simulink library "cps_lib_v2"  (R2012b)
settings: Solver=ode45  StartTime=0.0  StopTime=10.0  RelTol=1e-3
undefined symbols (not defined in the file or in its folder): block_height, block_mass, block_width, board_vpos, ini_block_hpos, ini_block_vpos, nozzle_radius
libraries: fl_lib x88, nesl_utility x7, vrlib x5, cps_physics_lib x3
settings Model: Creator=pmosterm  LastModifiedBy=pmosterm

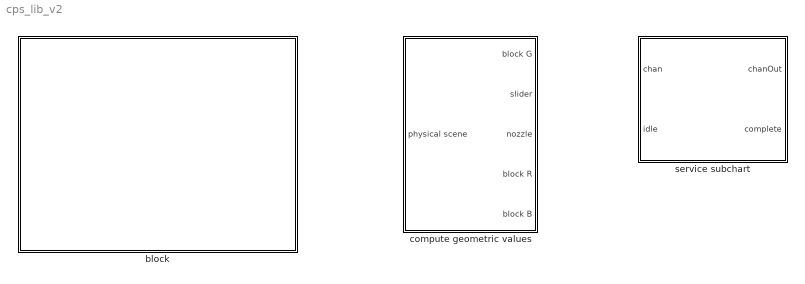
== system cps_lib_v2 ==
  block : Subsystem  mask{ini_block_vpos=ini_block_vpos, ini_block_hpos=ini_block_hpos}
      mask prompts: ini_block_vpos "Initial vertical block position"; ini_block_hpos "Initial horizontal block position"
      mask Display: image(imread('images\geo_ton_blocks_274x212.jpg'));
  compute geometric values : Subsystem
  service subchart : Stateflow chart  TreatAsAtomicUnit=on

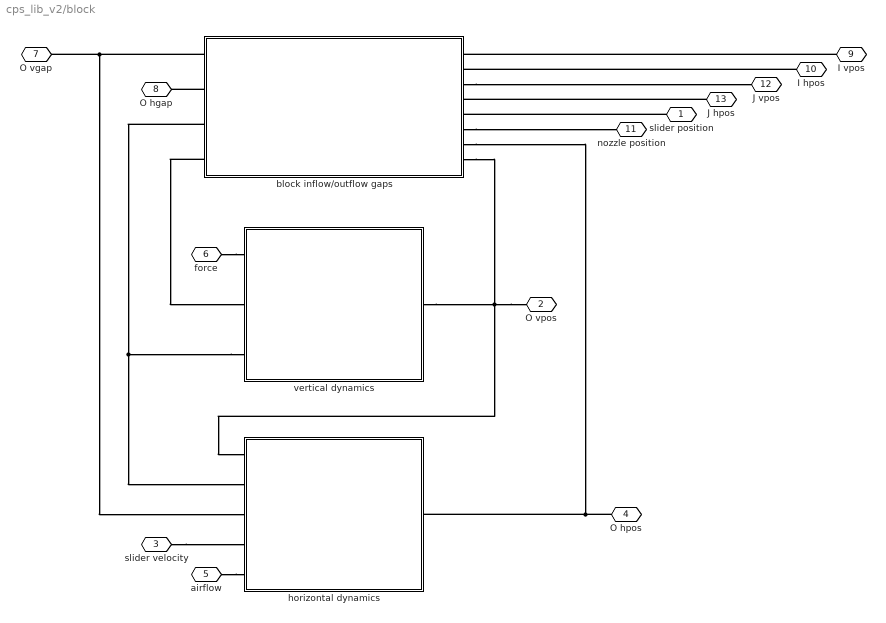
== system cps_lib_v2/block ==
  block inflow/outflow gaps : Subsystem
      settings: OpenFcn=open_system(gcb,'force');
      mask Display: image(imread('images\geo_ton_gaps_256x130.jpg'));
  horizontal dynamics : Subsystem
      settings: OpenFcn=open_system(gcb,'force');
      mask Display: image(imread('images\geo_ton_block_horizontal_176x149.jpg'));
  vertical dynamics : Subsystem
      settings: OpenFcn=open_system(gcb,'force');
      mask Display: image(imread('images\geo_ton_block_vertical_176x150.jpg'));
  slider position : PMIOPort  Port=1  Side=Left
  O vpos : PMIOPort  Port=2  Side=Right
  slider velocity : PMIOPort  Port=3  Side=Left
  O hpos : PMIOPort  Port=4  Side=Right
  airflow : PMIOPort  Port=5  Side=Left
  force : PMIOPort  Port=6  Side=Left
  O vgap : PMIOPort  Port=7  Side=Left
  O hgap : PMIOPort  Port=8  Side=Left
  I vpos : PMIOPort  Port=9  Side=Right
  I hpos : PMIOPort  Port=10  Side=Right
  nozzle position : PMIOPort  Port=11  Side=Left
  J vpos : PMIOPort  Port=12  Side=Right
  J hpos : PMIOPort  Port=13  Side=Right
  connections:
  block inflow/outflow gaps/LConn6 -- nozzle position/RConn1
  slider position/RConn1 -- block inflow/outflow gaps/LConn5
  I hpos/RConn1 -- block inflow/outflow gaps/LConn2
  I vpos/RConn1 -- block inflow/outflow gaps/LConn1
  block inflow/outflow gaps/RConn2 -- O hgap/RConn1
  block inflow/outflow gaps/RConn4 -- vertical dynamics/LConn2
  force/RConn1 -- vertical dynamics/LConn1
  vertical dynamics/LConn3 -- horizontal dynamics/LConn2 -- block inflow/outflow gaps/RConn3
  airflow/RConn1 -- horizontal dynamics/LConn5
  block inflow/outflow gaps/RConn1 -- horizontal dynamics/LConn3 -- O vgap/RConn1
  O vpos/RConn1 -- block inflow/outflow gaps/LConn8 -- horizontal dynamics/LConn1 -- vertical dynamics/RConn1
  horizontal dynamics/RConn1 -- block inflow/outflow gaps/LConn7 -- O hpos/RConn1
  slider velocity/RConn1 -- horizontal dynamics/LConn4
  block inflow/outflow gaps/LConn3 -- J vpos/RConn1
  J hpos/RConn1 -- block inflow/outflow gaps/LConn4

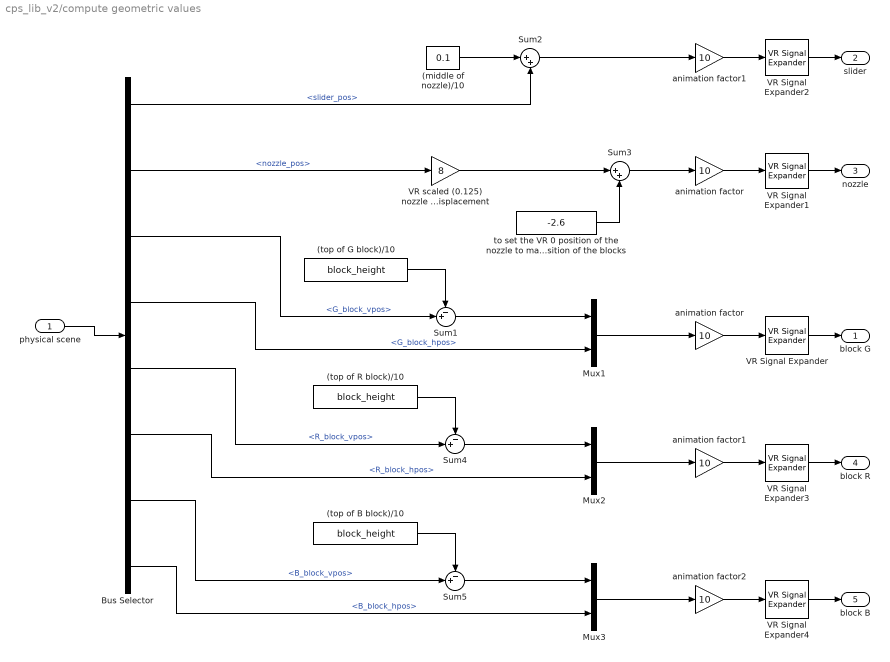
== system cps_lib_v2/compute geometric values ==
  physical scene : Inport  OutDataTypeStr=Bus: slBusGeometry
  " animation factor" : Gain  Gain=10
  " animation factor1" : Gain  Gain=10
  (middle of nozzle)/10 : Constant  Value=0.1
  (top of B block)/10 : Constant  Value=block_height
  (top of G block)/10 : Constant  Value=block_height
  (top of R block)/10 : Constant  Value=block_height
  Bus Selector : BusSelector  OutputSignals=slider_pos,nozzle_pos,G_block_vpos,G_block_hpos,R_block_vpos,R_block_hpos,B_block_vpos,B_block_hpos
  Mux1 : Mux  Inputs=2
  Mux2 : Mux  Inputs=2
  Mux3 : Mux  Inputs=2
  Sum1 : Sum  Inputs=-+|
  Sum2 : Sum  Inputs=|++
  Sum3 : Sum  Inputs=|++
  Sum4 : Sum  Inputs=-+|
  Sum5 : Sum  Inputs=-+|
  VR Signal Expander : vrlib/VR Signal Expander  outwidth=3  outidx=[2 3]
  VR Signal Expander1 : vrlib/VR Signal Expander  outwidth=3  outidx=[2]
  VR Signal Expander2 : vrlib/VR Signal Expander  outwidth=3  outidx=[3]
  VR Signal Expander3 : vrlib/VR Signal Expander  outwidth=3  outidx=[2 3]
  VR Signal Expander4 : vrlib/VR Signal Expander  outwidth=3  outidx=[2 3]
  VR scaled (0.125) nozzle displacement : Gain  Gain=8
  animation factor : Gain  Gain=10
  animation factor1 : Gain  Gain=10
  animation factor2 : Gain  Gain=10
  "to set the VR 0 position of the nozzle to match up with the VR 0 position of the blocks " : Constant  Value=-2.6
  block G : Outport
  slider : Outport  Port=2
  nozzle : Outport  Port=3
  block R : Outport  Port=4
  block B : Outport  Port=5
  wires:
  " animation factor"/1 -> VR Signal Expander1/1
  (middle of nozzle)/10/1 -> Sum2/1
  Bus Selector/1 -> Sum2/2  "<slider_pos>"
  animation factor/1 -> VR Signal Expander/1
  Mux1/1 -> animation factor/1
  Sum2/1 -> " animation factor1"/1
  VR Signal Expander2/1 -> slider/1
  VR Signal Expander1/1 -> nozzle/1
  Bus Selector/4 -> Mux1/2  "<G_block_hpos>"
  VR Signal Expander/1 -> block G/1
  " animation factor1"/1 -> VR Signal Expander2/1
  Sum3/1 -> " animation factor"/1
  Sum1/1 -> Mux1/1
  Bus Selector/3 -> Sum1/2  "<G_block_vpos>"
  Bus Selector/2 -> VR scaled (0.125) nozzle displacement/1  "<nozzle_pos>"
  physical scene/1 -> Bus Selector/1
  animation factor1/1 -> VR Signal Expander3/1
  Mux2/1 -> animation factor1/1
  VR Signal Expander3/1 -> block R/1
  Sum4/1 -> Mux2/1
  Bus Selector/6 -> Mux2/2  "<R_block_hpos>"
  Bus Selector/5 -> Sum4/2  "<R_block_vpos>"
  (top of G block)/10/1 -> Sum1/1
  (top of R block)/10/1 -> Sum4/1
  "to set the VR 0 position of the nozzle to match up with the VR 0 position of the blocks "/1 -> Sum3/2
  VR scaled (0.125) nozzle displacement/1 -> Sum3/1
  animation factor2/1 -> VR Signal Expander4/1
  Mux3/1 -> animation factor2/1
  VR Signal Expander4/1 -> block B/1
  Sum5/1 -> Mux3/1
  (top of B block)/10/1 -> Sum5/1
  Bus Selector/7 -> Sum5/2  "<B_block_vpos>"
  Bus Selector/8 -> Mux3/2  "<B_block_hpos>"

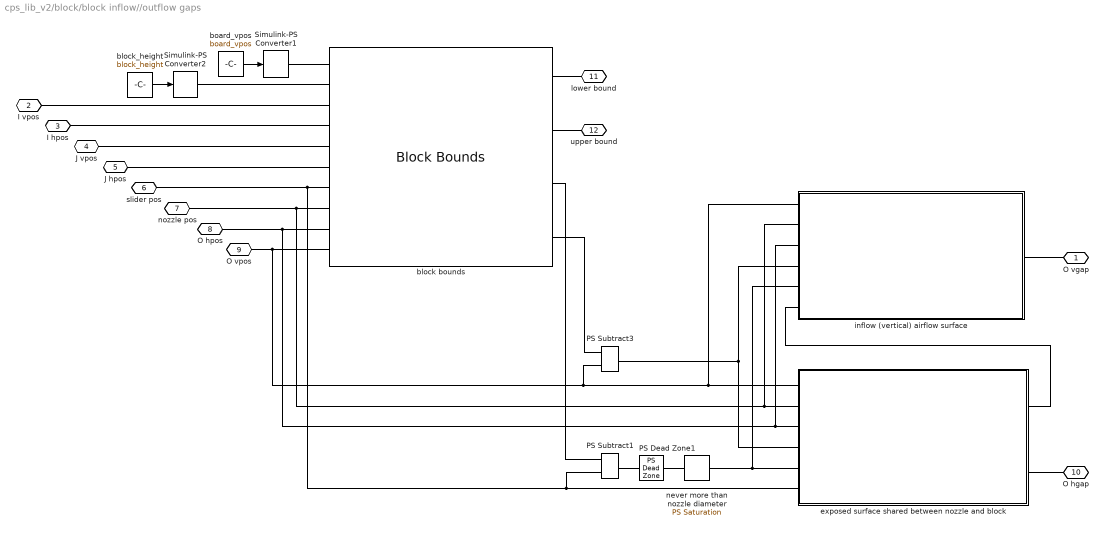
== system cps_lib_v2/block/block inflow//outflow gaps ==
  PS Dead Zone1 : fl_lib/Physical Signals/Nonlinear Operators/PS Dead Zone  upper_limit=0.5*block_width-nozzle_radius  lower_limit=-0.5*block_width+nozzle_radius  LocalVarLogging=[]
  PS Subtract1 : fl_lib/Physical Signals/Functions/PS Subtract  LocalVarLogging=[]
  PS Subtract3 : fl_lib/Physical Signals/Functions/PS Subtract  LocalVarLogging=[]
  Simulink-PS Converter1 : nesl_utility/Simulink-PS Converter  PhysicalDomain=network_engine_domain  LeftPortType=input  RightPortType=output  SubClassName=ps_input  PseudoPeriodic=off  Frequencies=[]  NoiseDistribution=none  NoiseParameters=[]  Unit=1  AffineConversion=off  InputFilterTimeConstant=.001  UdotUserProvided=[]  SimscapeFilterOrder=1  InputFiltering=off
  Simulink-PS Converter2 : nesl_utility/Simulink-PS Converter  PhysicalDomain=network_engine_domain  LeftPortType=input  RightPortType=output  SubClassName=ps_input  PseudoPeriodic=off  Frequencies=[]  NoiseDistribution=none  NoiseParameters=[]  Unit=1  AffineConversion=off  InputFilterTimeConstant=.001  UdotUserProvided=[]  SimscapeFilterOrder=1  InputFiltering=off
  block bounds : cps_physics_lib/Block Bounds  block_width=block_width m  nozzle_radius=nozzle_radius m  vmargin=1e-6 m  block_height_Log=off  board_vpos_Log=off  LocalVarNames=|block_height  LocalVarDescs=|Block Height  LocalVarLogging=[]
  block_height : Constant  Value=block_height
  board_vpos : Constant  Value=board_vpos
  exposed surface shared between nozzle and block : Subsystem
  inflow (vertical) airflow surface : Subsystem
  never more than nozzle diameter : fl_lib/Physical Signals/Nonlinear Operators/PS Saturation  upper_limit=2*nozzle_radius  lower_limit=-2*nozzle_radius  LocalVarLogging=[]
  O vgap : PMIOPort  Port=1  Side=Right
  I vpos : PMIOPort  Port=2  Side=Left
  I hpos : PMIOPort  Port=3  Side=Left
  J vpos : PMIOPort  Port=4  Side=Left
  J hpos : PMIOPort  Port=5  Side=Left
  slider pos : PMIOPort  Port=6  Side=Left
  nozzle pos : PMIOPort  Port=7  Side=Left
  O hpos : PMIOPort  Port=8  Side=Left
  O vpos : PMIOPort  Port=9  Side=Left
  O hgap : PMIOPort  Port=10  Side=Right
  lower bound : PMIOPort  Port=11  Side=Right
  upper bound : PMIOPort  Port=12  Side=Right
  wires:
  block_height/1 -> Simulink-PS Converter2/1
  board_vpos/1 -> Simulink-PS Converter1/1
  connections:
  PS Subtract1/RConn1 -- PS Dead Zone1/LConn1
  PS Dead Zone1/RConn1 -- never more than nozzle diameter/LConn1
  block bounds/LConn3 -- I vpos/RConn1
  never more than nozzle diameter/RConn1 -- exposed surface shared between nozzle and block/LConn5 -- inflow (vertical) airflow surface/LConn5
  block bounds/LConn4 -- I hpos/RConn1
  exposed surface shared between nozzle and block/LConn2 -- block bounds/LConn8 -- nozzle pos/RConn1 -- inflow (vertical) airflow surface/LConn2
  exposed surface shared between nozzle and block/LConn6 -- slider pos/RConn1 -- block bounds/LConn7 -- PS Subtract1/LConn2
  inflow (vertical) airflow surface/LConn1 -- exposed surface shared between nozzle and block/LConn1 -- block bounds/LConn10 -- O vpos/RConn1 -- PS Subtract3/LConn1
  inflow (vertical) airflow surface/LConn4 -- exposed surface shared between nozzle and block/LConn4 -- PS Subtract3/RConn1
  inflow (vertical) airflow surface/RConn1 -- O vgap/RConn1
  inflow (vertical) airflow surface/LConn3 -- exposed surface shared between nozzle and block/LConn3 -- block bounds/LConn9 -- O hpos/RConn1
  exposed surface shared between nozzle and block/RConn1 -- inflow (vertical) airflow surface/LConn6
  O hgap/RConn1 -- exposed surface shared between nozzle and block/RConn2
  block bounds/LConn5 -- J vpos/RConn1
  block bounds/LConn6 -- J hpos/RConn1
  block bounds/RConn1 -- lower bound/RConn1
  block bounds/RConn2 -- upper bound/RConn1
  block bounds/RConn4 -- PS Subtract3/LConn2
  block bounds/RConn3 -- PS Subtract1/LConn1
  Simulink-PS Converter2/RConn1 -- block bounds/LConn2
  Simulink-PS Converter1/RConn1 -- block bounds/LConn1

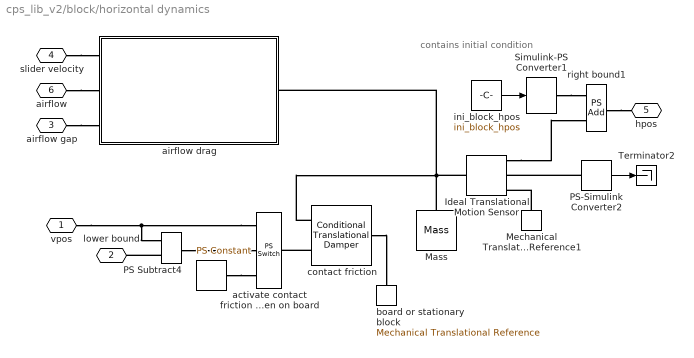
== system cps_lib_v2/block/horizontal dynamics ==
  note: contains initial condition
  " " : fl_lib/Physical Signals/Sources/PS Constant  constant=0  LocalVarLogging=[]
  Ideal Translational Motion Sensor : fl_lib/Mechanical/Mechanical Sensors/Ideal Translational Motion Sensor  offset=0 m  v_Log=off  f_Log=off  x_Log=off  LocalVarNames=|v|f|x  LocalVarDescs=|v|f|x  LocalVarLogging=[0 0 0]
  Mass : fl_lib/Mechanical/Translational Elements/Mass  mass=block_mass kg  initial_velocity=0 m/s  f_Log=off  LocalVarNames=|f  LocalVarDescs=|f  LocalVarLogging=0
  Mechanical Translational Reference1 : fl_lib/Mechanical/Translational Elements/Mechanical Translational Reference  f_Log=off  LocalVarNames=|f  LocalVarDescs=|f  LocalVarLogging=0
  PS Subtract4 : fl_lib/Physical Signals/Functions/PS Subtract  LocalVarLogging=[]
  PS-Simulink Converter2 : nesl_utility/PS-Simulink Converter  PhysicalDomain=network_engine_domain  LeftPortType=input  RightPortType=output  SubClassName=ps_output  PseudoPeriodic=off  Frequencies=[]  Unit=1  AffineConversion=off
  Simulink-PS Converter1 : nesl_utility/Simulink-PS Converter  PhysicalDomain=network_engine_domain  LeftPortType=input  RightPortType=output  SubClassName=ps_input  PseudoPeriodic=off  Frequencies=[]  NoiseDistribution=none  NoiseParameters=[]  Unit=1  AffineConversion=off  InputFilterTimeConstant=.001  UdotUserProvided=[]  SimscapeFilterOrder=1  InputFiltering=off
  Terminator2 : Terminator
  activate contact friction when on board : fl_lib/Physical Signals/Nonlinear Operators/PS Switch  Threshold=0  LocalVarLogging=[]
  airflow drag : Subsystem
  board or stationary block : fl_lib/Mechanical/Translational Elements/Mechanical Translational Reference  f_Log=off  LocalVarNames=|f  LocalVarDescs=|f  LocalVarLogging=0
  contact friction : cps_physics_lib/Conditional Translational Damper  D=100 N/(m/s)  th=1e-12  f_Log=off  v_Log=off  LocalVarNames=|f|v  LocalVarDescs=|f|v  LocalVarLogging=[0 0]
  ini_block_hpos : Constant  Value=ini_block_hpos
  right bound1 : fl_lib/Physical Signals/Functions/PS Add  LocalVarLogging=[]
  vpos : PMIOPort  Port=1  Side=Left
  lower bound : PMIOPort  Port=2  Side=Left
  airflow gap : PMIOPort  Port=3  Side=Left
  slider velocity : PMIOPort  Port=4  Side=Left
  hpos : PMIOPort  Port=5  Side=Right
  airflow : PMIOPort  Port=6  Side=Left
  wires:
  PS-Simulink Converter2/1 -> Terminator2/1
  ini_block_hpos/1 -> Simulink-PS Converter1/1
  connections:
  PS-Simulink Converter2/LConn1 -- Ideal Translational Motion Sensor/RConn2
  contact friction/LConn2 -- activate contact friction when on board/RConn1
  " "/RConn1 -- activate contact friction when on board/LConn3
  contact friction/RConn1 -- board or stationary block/LConn1
  PS Subtract4/RConn1 -- activate contact friction when on board/LConn2
  PS Subtract4/LConn2 -- lower bound/RConn1
  activate contact friction when on board/LConn1 -- vpos/RConn1 -- PS Subtract4/LConn1
  airflow gap/RConn1 -- airflow drag/LConn3
  airflow/RConn1 -- airflow drag/LConn2
  slider velocity/RConn1 -- airflow drag/LConn1
  Simulink-PS Converter1/RConn1 -- right bound1/LConn2
  Mechanical Translational Reference1/LConn1 -- Ideal Translational Motion Sensor/RConn1
  right bound1/RConn1 -- hpos/RConn1
  Ideal Translational Motion Sensor/RConn3 -- right bound1/LConn1
  Mass/LConn1 -- Ideal Translational Motion Sensor/LConn1 -- airflow drag/RConn1 -- contact friction/LConn1

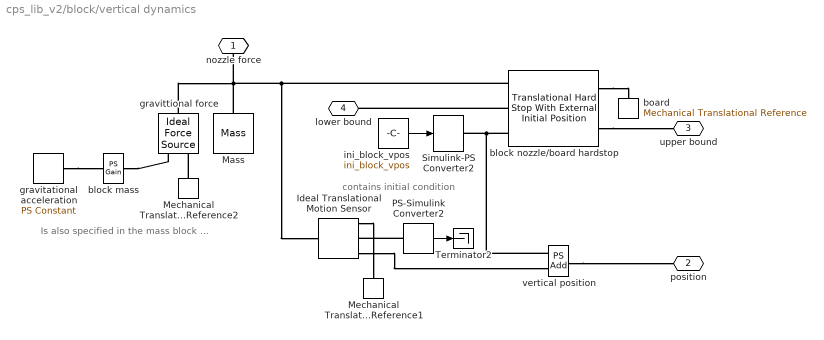
== system cps_lib_v2/block/vertical dynamics ==
  note: contains initial condition
  note: Is also specified in
      | the mass block ...
  Ideal Translational Motion Sensor : fl_lib/Mechanical/Mechanical Sensors/Ideal Translational Motion Sensor  offset=0 m  v_Log=off  f_Log=off  x_Log=off  LocalVarNames=|v|f|x  LocalVarDescs=|v|f|x  LocalVarLogging=[0 0 0]
  Mass : fl_lib/Mechanical/Translational Elements/Mass  mass=block_mass kg  initial_velocity=0 m/s  f_Log=off  LocalVarNames=|f  LocalVarDescs=|f  LocalVarLogging=0
  Mechanical Translational Reference1 : fl_lib/Mechanical/Translational Elements/Mechanical Translational Reference  f_Log=off  LocalVarNames=|f  LocalVarDescs=|f  LocalVarLogging=0
  Mechanical Translational Reference2 : fl_lib/Mechanical/Translational Elements/Mechanical Translational Reference  f_Log=off  LocalVarNames=|f  LocalVarDescs=|f  LocalVarLogging=0
  PS-Simulink Converter2 : nesl_utility/PS-Simulink Converter  PhysicalDomain=network_engine_domain  LeftPortType=input  RightPortType=output  SubClassName=ps_output  PseudoPeriodic=off  Frequencies=[]  Unit=1  AffineConversion=off
  Simulink-PS Converter2 : nesl_utility/Simulink-PS Converter  PhysicalDomain=network_engine_domain  LeftPortType=input  RightPortType=output  SubClassName=ps_input  PseudoPeriodic=off  Frequencies=[]  NoiseDistribution=none  NoiseParameters=[]  Unit=1  AffineConversion=off  InputFilterTimeConstant=.001  UdotUserProvided=[]  SimscapeFilterOrder=1  InputFiltering=off
  Terminator2 : Terminator
  block nozzle/board hardstop : cps_physics_lib/Translational Hard Stop With External Initial Position  stiff_up=3e4 N/m  stiff_low=1e5 N/m  D_up=450 N/(m/s)  D_low=450 N/(m/s)  f_Log=off  v_Log=off  x_Log=off  LocalVarNames=|f|v|x  LocalVarDescs=|f|v|x  LocalVarLogging=[0 0 0]
  block mass : fl_lib/Physical Signals/Functions/PS Gain  gain=block_mass  LocalVarLogging=[]
  board : fl_lib/Mechanical/Translational Elements/Mechanical Translational Reference  f_Log=off  LocalVarNames=|f  LocalVarDescs=|f  LocalVarLogging=0
  gravitational acceleration : fl_lib/Physical Signals/Sources/PS Constant  constant=-9.81  LocalVarLogging=[]
  gravittional force : fl_lib/Mechanical/Mechanical Sources/Ideal Force Source  v_Log=off  f_Log=off  LocalVarNames=|v|f  LocalVarDescs=|v|f  LocalVarLogging=[0 0]
  ini_block_vpos : Constant  Value=ini_block_vpos
  vertical position : fl_lib/Physical Signals/Functions/PS Add  LocalVarLogging=[]
  nozzle force : PMIOPort  Port=1  Side=Left
  position : PMIOPort  Port=2  Side=Right
  upper bound : PMIOPort  Port=3  Side=Left
  lower bound : PMIOPort  Port=4  Side=Left
  wires:
  PS-Simulink Converter2/1 -> Terminator2/1
  ini_block_vpos/1 -> Simulink-PS Converter2/1
  connections:
  PS-Simulink Converter2/LConn1 -- Ideal Translational Motion Sensor/RConn2
  Ideal Translational Motion Sensor/RConn3 -- vertical position/LConn2
  block nozzle/board hardstop/RConn2 -- upper bound/RConn1
  Simulink-PS Converter2/RConn1 -- block nozzle/board hardstop/LConn3 -- vertical position/LConn1
  block nozzle/board hardstop/RConn1 -- board/LConn1
  block nozzle/board hardstop/LConn2 -- lower bound/RConn1
  vertical position/RConn1 -- position/RConn1
  Ideal Translational Motion Sensor/RConn1 -- Mechanical Translational Reference1/LConn1
  nozzle force/RConn1 -- Mass/LConn1 -- gravittional force/LConn1 -- block nozzle/board hardstop/LConn1 -- Ideal Translational Motion Sensor/LConn1
  Mechanical Translational Reference2/LConn1 -- gravittional force/RConn2
  gravitational acceleration/RConn1 -- block mass/LConn1
  block mass/RConn1 -- gravittional force/RConn1

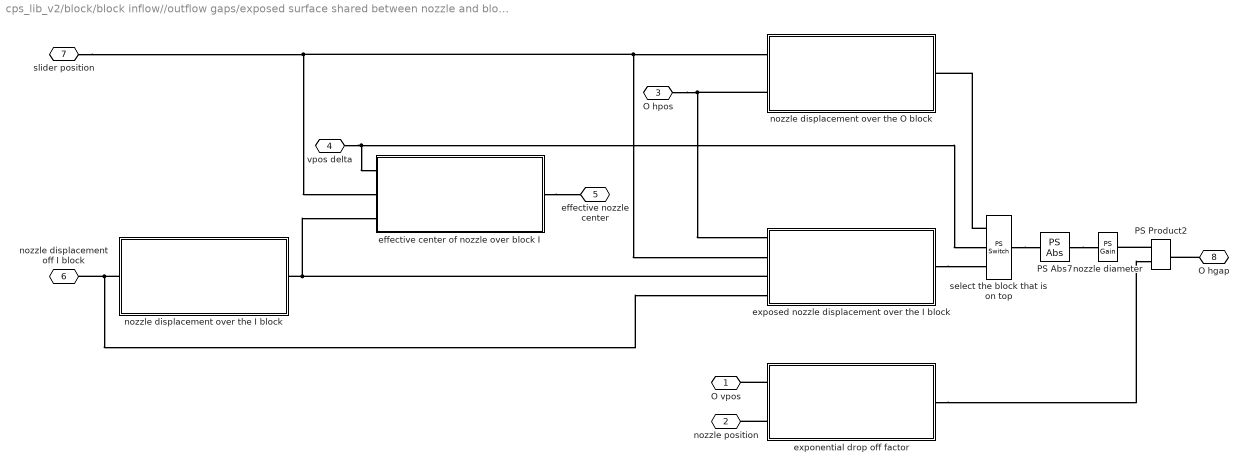
== system cps_lib_v2/block/block inflow//outflow gaps/exposed surface shared between nozzle and block ==
  PS Abs7 : fl_lib/Physical Signals/Nonlinear Operators/PS Abs  LocalVarLogging=[]
  PS Product2 : fl_lib/Physical Signals/Functions/PS Product  LocalVarLogging=[]
  effective center of nozzle over block I : Subsystem
  exponential drop off factor : Subsystem
  exposed nozzle displacement over the I block : Subsystem
  nozzle diameter : fl_lib/Physical Signals/Functions/PS Gain  gain=2*nozzle_radius  LocalVarLogging=[]
  nozzle displacement over the I block : Subsystem
  nozzle displacement over the O block : Subsystem
  select the block that is on top : fl_lib/Physical Signals/Nonlinear Operators/PS Switch  Threshold=0  LocalVarLogging=[]
  O vpos : PMIOPort  Port=1  Side=Left
  nozzle position : PMIOPort  Port=2  Side=Left
  O hpos : PMIOPort  Port=3  Side=Left
  vpos delta : PMIOPort  Port=4  Side=Left
  effective nozzle center : PMIOPort  Port=5  Side=Right
  nozzle displacement off I block : PMIOPort  Port=6  Side=Left
  slider position : PMIOPort  Port=7  Side=Left
  O hgap : PMIOPort  Port=8  Side=Right
  connections:
  select the block that is on top/RConn1 -- PS Abs7/LConn1
  O hgap/RConn1 -- PS Product2/RConn1
  PS Abs7/RConn1 -- nozzle diameter/LConn1
  PS Product2/LConn1 -- nozzle diameter/RConn1
  vpos delta/RConn1 -- select the block that is on top/LConn2 -- effective center of nozzle over block I/LConn1
  nozzle displacement over the I block/LConn1 -- nozzle displacement off I block/RConn1 -- exposed nozzle displacement over the I block/LConn4
  select the block that is on top/LConn1 -- nozzle displacement over the O block/RConn1
  exponential drop off factor/RConn1 -- PS Product2/LConn2
  exponential drop off factor/LConn1 -- O vpos/RConn1
  exponential drop off factor/LConn2 -- nozzle position/RConn1
  effective center of nozzle over block I/RConn1 -- effective nozzle center/RConn1
  slider position/RConn1 -- exposed nozzle displacement over the I block/LConn2 -- nozzle displacement over the O block/LConn1 -- effective center of nozzle over block I/LConn2
  exposed nozzle displacement over the I block/LConn3 -- nozzle displacement over the I block/RConn1 -- effective center of nozzle over block I/LConn3
  nozzle displacement over the O block/LConn2 -- exposed nozzle displacement over the I block/LConn1 -- O hpos/RConn1
  exposed nozzle displacement over the I block/RConn1 -- select the block that is on top/LConn3

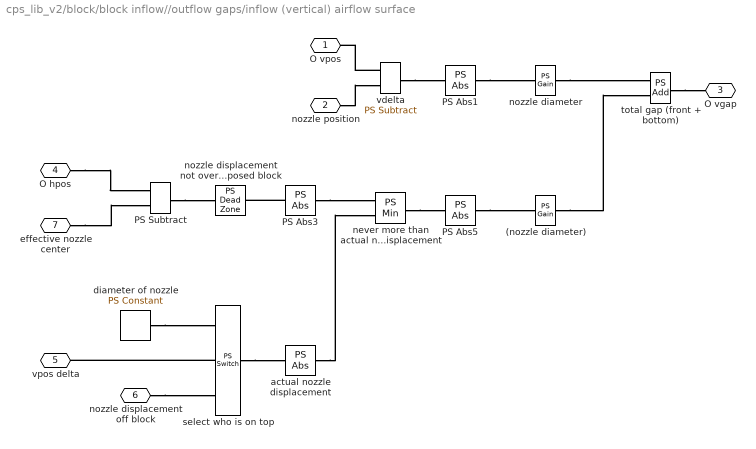
== system cps_lib_v2/block/block inflow//outflow gaps/inflow (vertical) airflow surface ==
  (nozzle diameter) : fl_lib/Physical Signals/Functions/PS Gain  gain=2*nozzle_radius  LocalVarLogging=[]
  PS Abs1 : fl_lib/Physical Signals/Nonlinear Operators/PS Abs  LocalVarLogging=[]
  PS Abs3 : fl_lib/Physical Signals/Nonlinear Operators/PS Abs  LocalVarLogging=[]
  PS Abs5 : fl_lib/Physical Signals/Nonlinear Operators/PS Abs  LocalVarLogging=[]
  PS Subtract : fl_lib/Physical Signals/Functions/PS Subtract  LocalVarLogging=[]
  actual nozzle displacement : fl_lib/Physical Signals/Nonlinear Operators/PS Abs  LocalVarLogging=[]
  diameter of nozzle : fl_lib/Physical Signals/Sources/PS Constant  constant=2*nozzle_radius  LocalVarLogging=[]
  never more than actual nozzle displacement : fl_lib/Physical Signals/Nonlinear Operators/PS Min  LocalVarLogging=[]
  nozzle diameter : fl_lib/Physical Signals/Functions/PS Gain  gain=2*nozzle_radius  LocalVarLogging=[]
  nozzle displacement not over exposed block : fl_lib/Physical Signals/Nonlinear Operators/PS Dead Zone  upper_limit=0.5*block_width-nozzle_radius  lower_limit=-0.5*block_width+nozzle_radius  LocalVarLogging=[]
  select who is on top : fl_lib/Physical Signals/Nonlinear Operators/PS Switch  Threshold=0  LocalVarLogging=[]
  total gap (front + bottom) : fl_lib/Physical Signals/Functions/PS Add  LocalVarLogging=[]
  vdelta : fl_lib/Physical Signals/Functions/PS Subtract  LocalVarLogging=[]
  O vpos : PMIOPort  Port=1  Side=Left
  nozzle position : PMIOPort  Port=2  Side=Left
  O vgap : PMIOPort  Port=3  Side=Right
  O hpos : PMIOPort  Port=4  Side=Left
  vpos delta : PMIOPort  Port=5  Side=Left
  nozzle displacement off block : PMIOPort  Port=6  Side=Left
  effective nozzle center : PMIOPort  Port=7  Side=Left
  connections:
  (nozzle diameter)/RConn1 -- total gap (front + bottom)/LConn2
  nozzle diameter/RConn1 -- total gap (front + bottom)/LConn1
  total gap (front + bottom)/RConn1 -- O vgap/RConn1
  PS Abs3/RConn1 -- never more than actual nozzle displacement/LConn1
  never more than actual nozzle displacement/RConn1 -- PS Abs5/LConn1
  select who is on top/RConn1 -- actual nozzle displacement/LConn1
  select who is on top/LConn2 -- vpos delta/RConn1
  PS Abs3/LConn1 -- nozzle displacement not over exposed block/RConn1
  PS Subtract/RConn1 -- nozzle displacement not over exposed block/LConn1
  PS Abs5/RConn1 -- (nozzle diameter)/LConn1
  diameter of nozzle/RConn1 -- select who is on top/LConn1
  vdelta/RConn1 -- PS Abs1/LConn1
  actual nozzle displacement/RConn1 -- never more than actual nozzle displacement/LConn2
  PS Abs1/RConn1 -- nozzle diameter/LConn1
  effective nozzle center/RConn1 -- PS Subtract/LConn2
  vdelta/LConn1 -- O vpos/RConn1
  O hpos/RConn1 -- PS Subtract/LConn1
  nozzle position/RConn1 -- vdelta/LConn2
  nozzle displacement off block/RConn1 -- select who is on top/LConn3

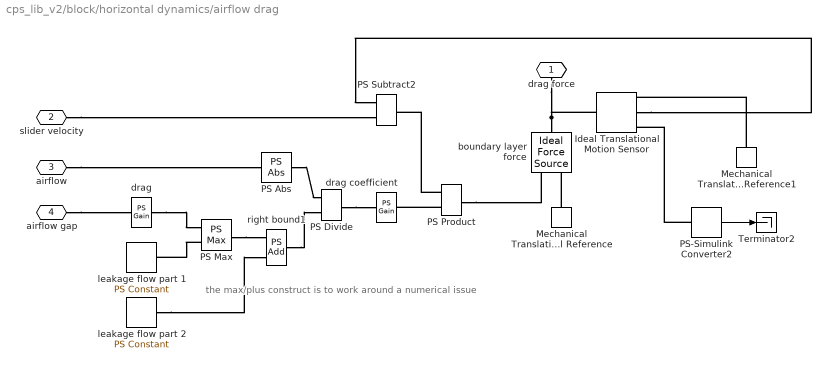
== system cps_lib_v2/block/horizontal dynamics/airflow drag ==
  note: the max/plus construct is to work
      | around a numerical issue
  Ideal Translational Motion Sensor : fl_lib/Mechanical/Mechanical Sensors/Ideal Translational Motion Sensor  offset=0 m  v_Log=off  f_Log=off  x_Log=off  LocalVarNames=|v|f|x  LocalVarDescs=|v|f|x  LocalVarLogging=[0 0 0]
  Mechanical Translational Reference : fl_lib/Mechanical/Translational Elements/Mechanical Translational Reference  f_Log=off  LocalVarNames=|f  LocalVarDescs=|f  LocalVarLogging=0
  Mechanical Translational Reference1 : fl_lib/Mechanical/Translational Elements/Mechanical Translational Reference  f_Log=off  LocalVarNames=|f  LocalVarDescs=|f  LocalVarLogging=0
  PS Abs : fl_lib/Physical Signals/Nonlinear Operators/PS Abs  LocalVarLogging=[]
  PS Divide : fl_lib/Physical Signals/Functions/PS Divide  LocalVarLogging=[]
  PS Max : fl_lib/Physical Signals/Nonlinear Operators/PS Max  LocalVarLogging=[]
  PS Product : fl_lib/Physical Signals/Functions/PS Product  LocalVarLogging=[]
  PS Subtract2 : fl_lib/Physical Signals/Functions/PS Subtract  LocalVarLogging=[]
  PS-Simulink Converter2 : nesl_utility/PS-Simulink Converter  PhysicalDomain=network_engine_domain  LeftPortType=input  RightPortType=output  SubClassName=ps_output  PseudoPeriodic=off  Frequencies=[]  Unit=1  AffineConversion=off
  Terminator2 : Terminator
  boundary layer force : fl_lib/Mechanical/Mechanical Sources/Ideal Force Source  v_Log=off  f_Log=off  LocalVarNames=|v|f  LocalVarDescs=|v|f  LocalVarLogging=[0 0]
  drag : fl_lib/Physical Signals/Functions/PS Gain  gain=25  LocalVarLogging=[]
  drag coefficient : fl_lib/Physical Signals/Functions/PS Gain  gain=10.75e-1  LocalVarLogging=[]
  leakage flow part 1 : fl_lib/Physical Signals/Sources/PS Constant  constant=20e-3  LocalVarLogging=[]
  leakage flow part 2 : fl_lib/Physical Signals/Sources/PS Constant  constant=5e-3  LocalVarLogging=[]
  right bound1 : fl_lib/Physical Signals/Functions/PS Add  LocalVarLogging=[]
  drag force : PMIOPort  Port=1  Side=Right
  slider velocity : PMIOPort  Port=2  Side=Left
  airflow : PMIOPort  Port=3  Side=Left
  airflow gap : PMIOPort  Port=4  Side=Left
  wires:
  PS-Simulink Converter2/1 -> Terminator2/1
  connections:
  PS-Simulink Converter2/LConn1 -- Ideal Translational Motion Sensor/RConn3
  Mechanical Translational Reference1/LConn1 -- Ideal Translational Motion Sensor/RConn1
  boundary layer force/LConn1 -- Ideal Translational Motion Sensor/LConn1 -- drag force/RConn1
  Ideal Translational Motion Sensor/RConn2 -- PS Subtract2/LConn2
  PS Abs/RConn1 -- PS Divide/LConn1
  PS Product/LConn2 -- drag coefficient/RConn1
  Mechanical Translational Reference/LConn1 -- boundary layer force/RConn2
  PS Product/RConn1 -- boundary layer force/RConn1
  airflow gap/RConn1 -- drag/LConn1
  drag/RConn1 -- PS Max/LConn1
  slider velocity/RConn1 -- PS Subtract2/LConn1
  airflow/RConn1 -- PS Abs/LConn1
  PS Product/LConn1 -- PS Subtract2/RConn1
  PS Divide/RConn1 -- drag coefficient/LConn1
  PS Max/LConn2 -- leakage flow part 1/RConn1
  PS Max/RConn1 -- right bound1/LConn2
  right bound1/RConn1 -- PS Divide/LConn2
  leakage flow part 2/RConn1 -- right bound1/LConn1

== system cps_lib_v2/block/block inflow//outflow gaps/exposed surface shared between nozzle and block/effective center of nozzle over block I ==
  PS Add3 : fl_lib/Physical Signals/Functions/PS Add  LocalVarLogging=[]
  select effective nozzle center : fl_lib/Physical Signals/Nonlinear Operators/PS Switch  Threshold=0  LocalVarLogging=[]
  is block I on top : PMIOPort  Port=1  Side=Left
  nozzle center : PMIOPort  Port=2  Side=Left
  effective center : PMIOPort  Port=3  Side=Right
  displacement over block : PMIOPort  Port=4  Side=Left
  connections:
  PS Add3/LConn2 -- displacement over block/RConn1
  select effective nozzle center/RConn1 -- effective center/RConn1
  PS Add3/RConn1 -- select effective nozzle center/LConn3
  is block I on top/RConn1 -- select effective nozzle center/LConn2
  PS Add3/LConn1 -- nozzle center/RConn1 -- select effective nozzle center/LConn1

== system cps_lib_v2/block/block inflow//outflow gaps/exposed surface shared between nozzle and block/exponential drop off factor ==
  block/nozzle delta : fl_lib/Physical Signals/Functions/PS Subtract  LocalVarLogging=[]
  exp(u) : fl_lib/Physical Signals/Functions/PS Math Function  fcn_choice=3  LocalVarLogging=[]
  exponential drop-off factor : fl_lib/Physical Signals/Functions/PS Gain  gain=20  LocalVarLogging=[]
  drop off : PMIOPort  Port=1  Side=Right
  O vpos : PMIOPort  Port=2  Side=Left
  nozzle pos : PMIOPort  Port=3  Side=Left
  connections:
  exponential drop-off factor/RConn1 -- exp(u)/LConn1
  block/nozzle delta/RConn1 -- exponential drop-off factor/LConn1
  block/nozzle delta/LConn2 -- nozzle pos/RConn1
  exp(u)/RConn1 -- drop off/RConn1
  block/nozzle delta/LConn1 -- O vpos/RConn1

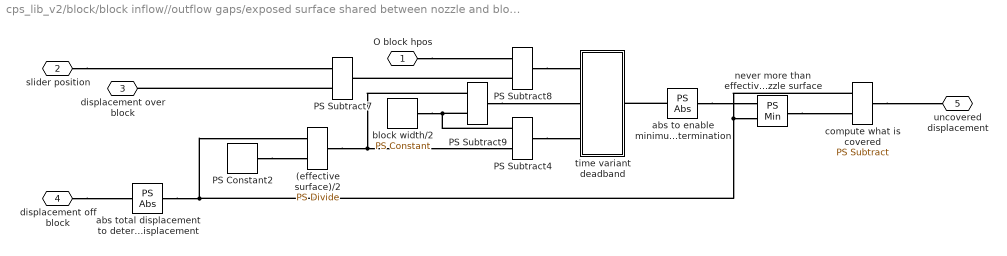
== system cps_lib_v2/block/block inflow//outflow gaps/exposed surface shared between nozzle and block/exposed nozzle displacement over the I block ==
  (effective surface)/2 : fl_lib/Physical Signals/Functions/PS Divide  LocalVarLogging=[]
  PS Constant2 : fl_lib/Physical Signals/Sources/PS Constant  constant=2  LocalVarLogging=[]
  PS Subtract{4,7..9} (4 alike) : fl_lib/Physical Signals/Functions/PS Subtract  LocalVarLogging=[]
  abs to enable minimum determination : fl_lib/Physical Signals/Nonlinear Operators/PS Abs  LocalVarLogging=[]
  abs total displacement to determine minimum with effective nozzle displacement : fl_lib/Physical Signals/Nonlinear Operators/PS Abs  LocalVarLogging=[]
  block width/2 : fl_lib/Physical Signals/Sources/PS Constant  constant=block_width/2  LocalVarLogging=[]
  compute what is covered : fl_lib/Physical Signals/Functions/PS Subtract  LocalVarLogging=[]
  never more than effective nozzle surface : fl_lib/Physical Signals/Nonlinear Operators/PS Min  LocalVarLogging=[]
  time variant deadband : Subsystem
  O block hpos : PMIOPort  Port=1  Side=Left
  slider position : PMIOPort  Port=2  Side=Left
  displacement over block : PMIOPort  Port=3  Side=Left
  displacement off block : PMIOPort  Port=4  Side=Left
  uncovered displacement : PMIOPort  Port=5  Side=Right
  connections:
  slider position/RConn1 -- PS Subtract7/LConn1
  displacement off block/RConn1 -- abs total displacement to determine minimum with effective nozzle displacement/LConn1
  O block hpos/RConn1 -- PS Subtract8/LConn1
  PS Subtract9/LConn1 -- (effective surface)/2/RConn1 -- PS Subtract4/LConn2
  compute what is covered/LConn1 -- (effective surface)/2/LConn1 -- abs total displacement to determine minimum with effective nozzle displacement/RConn1 -- never more than effective nozzle surface/LConn2
  PS Subtract9/RConn1 -- time variant deadband/LConn2
  PS Constant2/RConn1 -- (effective surface)/2/LConn2
  compute what is covered/RConn1 -- uncovered displacement/RConn1
  never more than effective nozzle surface/RConn1 -- compute what is covered/LConn2
  block width/2/RConn1 -- PS Subtract9/LConn2 -- PS Subtract4/LConn1
  PS Subtract8/LConn2 -- PS Subtract7/RConn1
  abs to enable minimum determination/RConn1 -- never more than effective nozzle surface/LConn1
  PS Subtract8/RConn1 -- time variant deadband/LConn1
  PS Subtract4/RConn1 -- time variant deadband/LConn3
  abs to enable minimum determination/LConn1 -- time variant deadband/RConn1
  PS Subtract7/LConn2 -- displacement over block/RConn1

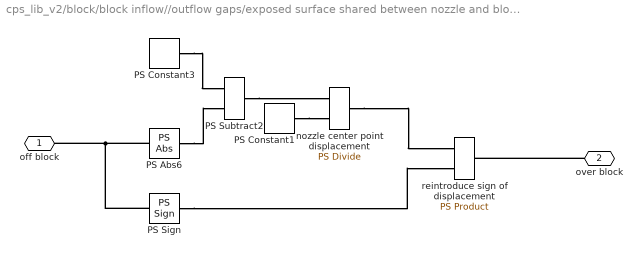
== system cps_lib_v2/block/block inflow//outflow gaps/exposed surface shared between nozzle and block/nozzle displacement over the I block ==
  PS Abs6 : fl_lib/Physical Signals/Nonlinear Operators/PS Abs  LocalVarLogging=[]
  PS Constant1 : fl_lib/Physical Signals/Sources/PS Constant  constant=2  LocalVarLogging=[]
  PS Constant3 : fl_lib/Physical Signals/Sources/PS Constant  constant=block_width  LocalVarLogging=[]
  PS Sign : fl_lib/Physical Signals/Nonlinear Operators/PS Sign  LocalVarLogging=[]
  PS Subtract2 : fl_lib/Physical Signals/Functions/PS Subtract  LocalVarLogging=[]
  nozzle center point displacement : fl_lib/Physical Signals/Functions/PS Divide  LocalVarLogging=[]
  reintroduce sign of displacement : fl_lib/Physical Signals/Functions/PS Product  LocalVarLogging=[]
  off block : PMIOPort  Port=1  Side=Left
  over block : PMIOPort  Port=2  Side=Right
  connections:
  PS Sign/LConn1 -- PS Abs6/LConn1 -- off block/RConn1
  over block/RConn1 -- reintroduce sign of displacement/RConn1
  PS Constant1/RConn1 -- nozzle center point displacement/LConn2
  PS Abs6/RConn1 -- PS Subtract2/LConn2
  PS Constant3/RConn1 -- PS Subtract2/LConn1
  PS Sign/RConn1 -- reintroduce sign of displacement/LConn2
  PS Subtract2/RConn1 -- nozzle center point displacement/LConn1
  nozzle center point displacement/RConn1 -- reintroduce sign of displacement/LConn1

== system cps_lib_v2/block/block inflow//outflow gaps/exposed surface shared between nozzle and block/nozzle displacement over the O block ==
  PS Abs2 : fl_lib/Physical Signals/Nonlinear Operators/PS Abs  LocalVarLogging=[]
  PS Constant7 : fl_lib/Physical Signals/Sources/PS Constant  constant=2*nozzle_radius  LocalVarLogging=[]
  PS Subtract5 : fl_lib/Physical Signals/Functions/PS Subtract  LocalVarLogging=[]
  maximum displacement is the nozzle radius : fl_lib/Physical Signals/Nonlinear Operators/PS Saturation  upper_limit=2*nozzle_radius  lower_limit=0  LocalVarLogging=[]
  nozzle displacement not over block : fl_lib/Physical Signals/Nonlinear Operators/PS Dead Zone  upper_limit=0.5*block_width-nozzle_radius  lower_limit=-0.5*block_width+nozzle_radius  LocalVarLogging=[]
  nozzle displacement that is over the block : fl_lib/Physical Signals/Functions/PS Subtract  LocalVarLogging=[]
  nozzle hpos : PMIOPort  Port=1  Side=Left
  block hpos : PMIOPort  Port=2  Side=Left
  effective displacement : PMIOPort  Port=3  Side=Right
  connections:
  PS Constant7/RConn1 -- nozzle displacement that is over the block/LConn1
  PS Subtract5/RConn1 -- nozzle displacement not over block/LConn1
  effective displacement/RConn1 -- nozzle displacement that is over the block/RConn1
  maximum displacement is the nozzle radius/RConn1 -- nozzle displacement that is over the block/LConn2
  nozzle displacement not over block/RConn1 -- PS Abs2/LConn1
  PS Abs2/RConn1 -- maximum displacement is the nozzle radius/LConn1
  PS Subtract5/LConn2 -- nozzle hpos/RConn1
  PS Subtract5/LConn1 -- block hpos/RConn1

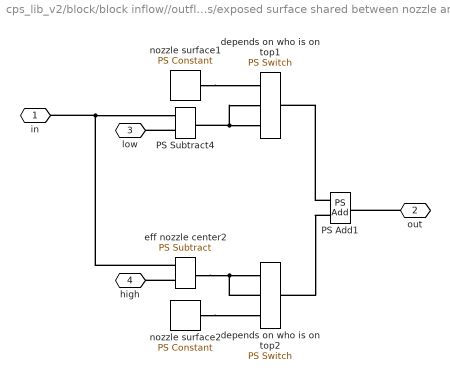
== system cps_lib_v2/block/block inflow//outflow gaps/exposed surface shared between nozzle and block/exposed nozzle displacement over the I block/time variant deadband ==
  PS Add1 : fl_lib/Physical Signals/Functions/PS Add  LocalVarLogging=[]
  PS Subtract4 : fl_lib/Physical Signals/Functions/PS Subtract  LocalVarLogging=[]
  depends on who is on top1 : fl_lib/Physical Signals/Nonlinear Operators/PS Switch  Threshold=0  LocalVarLogging=[]
  depends on who is on top2 : fl_lib/Physical Signals/Nonlinear Operators/PS Switch  Threshold=0  LocalVarLogging=[]
  eff nozzle center2 : fl_lib/Physical Signals/Functions/PS Subtract  LocalVarLogging=[]
  nozzle surface1 : fl_lib/Physical Signals/Sources/PS Constant  constant=0  LocalVarLogging=[]
  nozzle surface2 : fl_lib/Physical Signals/Sources/PS Constant  constant=0  LocalVarLogging=[]
  in : PMIOPort  Port=1  Side=Left
  out : PMIOPort  Port=2  Side=Right
  low : PMIOPort  Port=3  Side=Left
  high : PMIOPort  Port=4  Side=Left
  connections:
  eff nozzle center2/LConn2 -- high/RConn1
  PS Subtract4/LConn2 -- low/RConn1
  eff nozzle center2/LConn1 -- PS Subtract4/LConn1 -- in/RConn1
  depends on who is on top2/LConn2 -- depends on who is on top2/LConn1 -- eff nozzle center2/RConn1
  PS Add1/LConn1 -- depends on who is on top1/RConn1
  nozzle surface2/RConn1 -- depends on who is on top2/LConn3
  PS Add1/LConn2 -- depends on who is on top2/RConn1
  PS Subtract4/RConn1 -- depends on who is on top1/LConn3 -- depends on who is on top1/LConn2
  nozzle surface1/RConn1 -- depends on who is on top1/LConn1
  out/RConn1 -- PS Add1/RConn1

== stateflow chart cps_lib_v2/service subchart ==
  state action
    en: chanOut = chan.moveBlock;
  note: Need this sync state to
      | ensure an operation is
      | actually started before
      | considering complete again
  state sync
    ex: chanOut.move = 0;
  note: If you do not reset the
      | move operation, the
      | super goes straight into
      | a new operation
  state neutral
    du: complete = true;
  (default) -> action
  action -> sync : [~idle]
  sync -> neutral : [idle]
  data: chan input; idle input; chanOut output Bus: slBusMoveBlock; complete output double
